simulink model "SmartAgroSense"  (R2026a)
settings: Solver=FixedStepAuto  StopTime=100  FixedStep=0.1
settings Model: Creator=rasul  LastModifiedBy=rasul

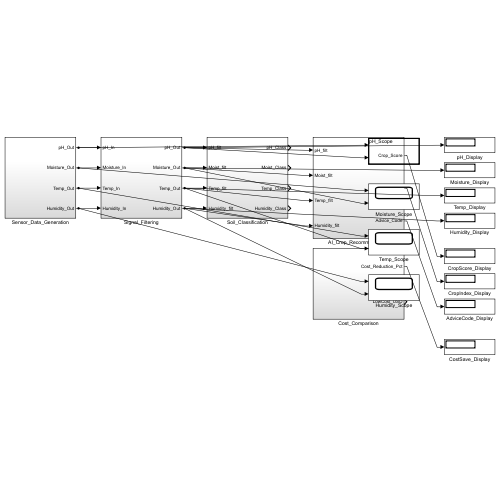
[thumbnail: Simulink's stored preview of the top-level diagram]
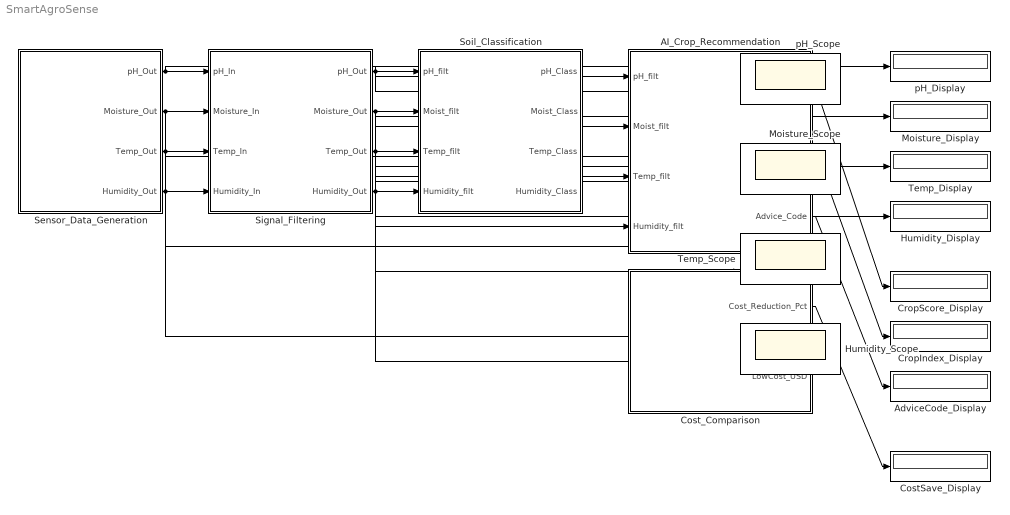
== system SmartAgroSense ==
  AI_Crop_Recommendation : Subsystem
  AdviceCode_Display : Display
  CostSave_Display : Display
  Cost_Comparison : Subsystem
  CropIndex_Display : Display
  CropScore_Display : Display
  Humidity_Display : Display
  Humidity_Scope : Scope  NumInputPorts=2
  Moisture_Display : Display
  Moisture_Scope : Scope  NumInputPorts=2
  Sensor_Data_Generation : Subsystem
  Signal_Filtering : Subsystem
  Soil_Classification : Subsystem
  Temp_Display : Display
  Temp_Scope : Scope  NumInputPorts=2
  pH_Display : Display
  pH_Scope : Scope  NumInputPorts=2
  wires:
  Sensor_Data_Generation/1(pH_Out) -> Signal_Filtering/1(pH_In), pH_Scope/1
  Sensor_Data_Generation/2(Moisture_Out) -> Signal_Filtering/2(Moisture_In), Moisture_Scope/1
  Sensor_Data_Generation/3(Temp_Out) -> Signal_Filtering/3(Temp_In), Temp_Scope/1
  Sensor_Data_Generation/4(Humidity_Out) -> Signal_Filtering/4(Humidity_In), Humidity_Scope/1
  Signal_Filtering/1(pH_Out) -> Soil_Classification/1(pH_filt), AI_Crop_Recommendation/1(pH_filt), pH_Display/1, pH_Scope/2
  Signal_Filtering/2(Moisture_Out) -> Soil_Classification/2(Moist_filt), AI_Crop_Recommendation/2(Moist_filt), Moisture_Display/1, Moisture_Scope/2
  Signal_Filtering/3(Temp_Out) -> Soil_Classification/3(Temp_filt), AI_Crop_Recommendation/3(Temp_filt), Temp_Display/1, Temp_Scope/2
  Signal_Filtering/4(Humidity_Out) -> Soil_Classification/4(Humidity_filt), AI_Crop_Recommendation/4(Humidity_filt), Humidity_Display/1, Humidity_Scope/2
  AI_Crop_Recommendation/1(Crop_Score) -> CropScore_Display/1
  AI_Crop_Recommendation/2(Crop_Index) -> CropIndex_Display/1
  AI_Crop_Recommendation/3(Advice_Code) -> AdviceCode_Display/1
  Cost_Comparison/1(Cost_Reduction_Pct) -> CostSave_Display/1

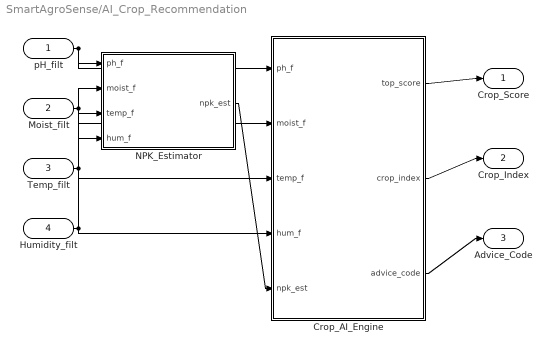
== system SmartAgroSense/AI_Crop_Recommendation ==
  pH_filt : Inport
  Moist_filt : Inport  Port=2
  Temp_filt : Inport  Port=3
  Humidity_filt : Inport  Port=4
  Crop_AI_Engine : MATLAB Function  TreatAsAtomicUnit=on
  NPK_Estimator : MATLAB Function  TreatAsAtomicUnit=on
  Crop_Score : Outport
  Crop_Index : Outport  Port=2
  Advice_Code : Outport  Port=3
  wires:
  pH_filt/1 -> Crop_AI_Engine/1(ph_f), NPK_Estimator/1(ph_f)
  Moist_filt/1 -> Crop_AI_Engine/2(moist_f), NPK_Estimator/2(moist_f)
  Temp_filt/1 -> Crop_AI_Engine/3(temp_f), NPK_Estimator/3(temp_f)
  Humidity_filt/1 -> Crop_AI_Engine/4(hum_f), NPK_Estimator/4(hum_f)
  NPK_Estimator/1(npk_est) -> Crop_AI_Engine/5(npk_est)
  Crop_AI_Engine/1(top_score) -> Crop_Score/1
  Crop_AI_Engine/2(crop_index) -> Crop_Index/1
  Crop_AI_Engine/3(advice_code) -> Advice_Code/1

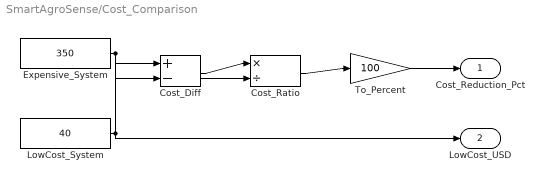
== system SmartAgroSense/Cost_Comparison ==
  Cost_Diff : Sum  Inputs=+-
  Cost_Ratio : Product  Inputs=*/
  Expensive_System : Constant  Value=350
  LowCost_System : Constant  Value=40
  To_Percent : Gain  Gain=100
  Cost_Reduction_Pct : Outport
  LowCost_USD : Outport  Port=2
  wires:
  Expensive_System/1 -> Cost_Diff/1, Cost_Ratio/2
  LowCost_System/1 -> Cost_Diff/2, LowCost_USD/1
  Cost_Diff/1 -> Cost_Ratio/1
  Cost_Ratio/1 -> To_Percent/1
  To_Percent/1 -> Cost_Reduction_Pct/1

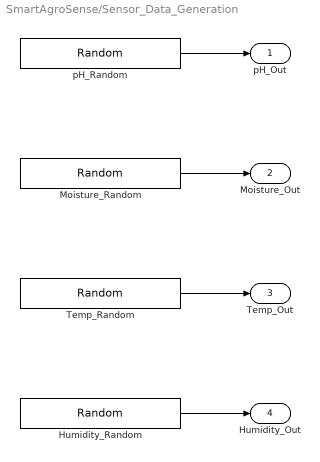
== system SmartAgroSense/Sensor_Data_Generation ==
  Humidity_Random : UniformRandomNumber  Minimum=30  Maximum=95  Seed=1088592771  SampleTime=0.1
  Moisture_Random : UniformRandomNumber  Minimum=10  Maximum=90  Seed=846067018  SampleTime=0.1
  Temp_Random : UniformRandomNumber  Minimum=10  Maximum=40  Seed=366663745  SampleTime=0.1
  pH_Random : UniformRandomNumber  Minimum=4.5  Maximum=8.5  Seed=1463581336  SampleTime=0.1
  pH_Out : Outport
  Moisture_Out : Outport  Port=2
  Temp_Out : Outport  Port=3
  Humidity_Out : Outport  Port=4
  wires:
  pH_Random/1 -> pH_Out/1
  Moisture_Random/1 -> Moisture_Out/1
  Temp_Random/1 -> Temp_Out/1
  Humidity_Random/1 -> Humidity_Out/1

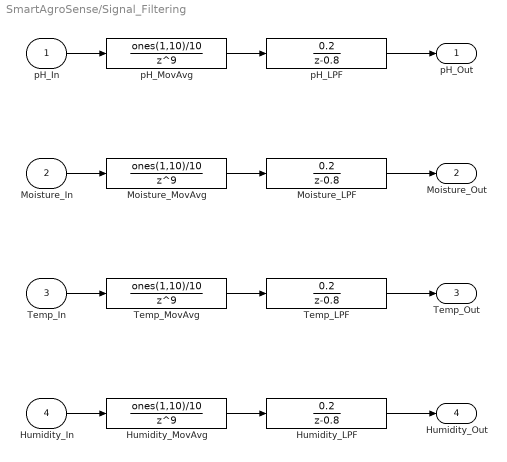
== system SmartAgroSense/Signal_Filtering ==
  pH_In : Inport
  Moisture_In : Inport  Port=2
  Temp_In : Inport  Port=3
  Humidity_In : Inport  Port=4
  Humidity_LPF : DiscreteTransferFcn  Numerator=[0.2]  Denominator=[1, -0.8]  SampleTime=0.1
  Humidity_MovAvg : DiscreteTransferFcn  Numerator=ones(1,10)/10  Denominator=[1 0 0 0 0 0 0 0 0 0]  SampleTime=0.1
  Moisture_LPF : DiscreteTransferFcn  Numerator=[0.2]  Denominator=[1, -0.8]  SampleTime=0.1
  Moisture_MovAvg : DiscreteTransferFcn  Numerator=ones(1,10)/10  Denominator=[1 0 0 0 0 0 0 0 0 0]  SampleTime=0.1
  Temp_LPF : DiscreteTransferFcn  Numerator=[0.2]  Denominator=[1, -0.8]  SampleTime=0.1
  Temp_MovAvg : DiscreteTransferFcn  Numerator=ones(1,10)/10  Denominator=[1 0 0 0 0 0 0 0 0 0]  SampleTime=0.1
  pH_LPF : DiscreteTransferFcn  Numerator=[0.2]  Denominator=[1, -0.8]  SampleTime=0.1
  pH_MovAvg : DiscreteTransferFcn  Numerator=ones(1,10)/10  Denominator=[1 0 0 0 0 0 0 0 0 0]  SampleTime=0.1
  pH_Out : Outport
  Moisture_Out : Outport  Port=2
  Temp_Out : Outport  Port=3
  Humidity_Out : Outport  Port=4
  wires:
  pH_In/1 -> pH_MovAvg/1
  pH_MovAvg/1 -> pH_LPF/1
  pH_LPF/1 -> pH_Out/1
  Moisture_In/1 -> Moisture_MovAvg/1
  Moisture_MovAvg/1 -> Moisture_LPF/1
  Moisture_LPF/1 -> Moisture_Out/1
  Temp_In/1 -> Temp_MovAvg/1
  Temp_MovAvg/1 -> Temp_LPF/1
  Temp_LPF/1 -> Temp_Out/1
  Humidity_In/1 -> Humidity_MovAvg/1
  Humidity_MovAvg/1 -> Humidity_LPF/1
  Humidity_LPF/1 -> Humidity_Out/1

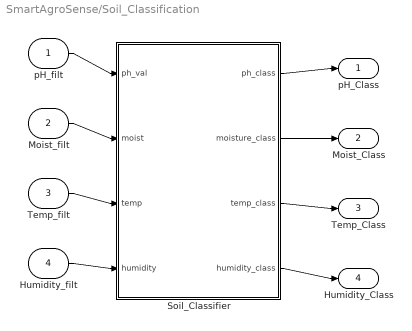
== system SmartAgroSense/Soil_Classification ==
  pH_filt : Inport
  Moist_filt : Inport  Port=2
  Temp_filt : Inport  Port=3
  Humidity_filt : Inport  Port=4
  Soil_Classifier : MATLAB Function  TreatAsAtomicUnit=on
  pH_Class : Outport
  Moist_Class : Outport  Port=2
  Temp_Class : Outport  Port=3
  Humidity_Class : Outport  Port=4
  wires:
  pH_filt/1 -> Soil_Classifier/1(ph_val)
  Moist_filt/1 -> Soil_Classifier/2(moist)
  Temp_filt/1 -> Soil_Classifier/3(temp)
  Humidity_filt/1 -> Soil_Classifier/4(humidity)
  Soil_Classifier/1(ph_class) -> pH_Class/1
  Soil_Classifier/2(moisture_class) -> Moist_Class/1
  Soil_Classifier/3(temp_class) -> Temp_Class/1
  Soil_Classifier/4(humidity_class) -> Humidity_Class/1

== matlab function SmartAgroSense/AI_Crop_Recommendation/NPK_Estimator ==
  data: ph_f input; npk_est output; moist_f input; temp_f input; hum_f input
%% =========================================================================
%  MATLAB Function Block: NPK_Estimator
%  File: npk_estimator_fcn.m
%
%  PURPOSE:
%    Estimate composite NPK availability score (0-100) from filtered
%    pH, moisture, temperature, and humidity readings.
%
%  INPUTS:
%    ph_f    - Filtered pH (4.5 to 8.5)
%    moist_f - Filtered soil moisture % (10 to 90)
%    temp_f  - Filtered temperature C (10 to 40)
%    hum_f   - Filtered humidity % (30 to 95)
%
%  OUTPUT:
%    npk_est - Composite NPK estimate (0 to 100)
%
%  PASTE THIS CODE INTO THE MATLAB FUNCTION BLOCK EDITOR IN SIMULINK
% =========================================================================

function npk_est = npk_estimator(ph_f, moist_f, temp_f, hum_f)
%#codegen

% NPK estimation heuristic:
% - pH near 6.5 generally improves nutrient availability
% - moderate moisture supports uptake
% - temperature/humidity adjust estimated N/P/K availability
ph_penalty = max(0, 1 - abs(ph_f - 6.5) / 2.0);           % 0-1
moist_factor = min(1, max(0, (moist_f - 20) / 50));       % 0-1
temp_factor = max(0, 1 - abs(temp_f - 24) / 16);          % 0-1
hum_factor = min(1, max(0, (hum_f - 35) / 45));           % 0-1

npk_base = 100 * (0.6 * ph_penalty + 0.4 * moist_factor);

n_est = npk_base * (0.85 + 0.25 * moist_factor - 0.10 * (1 - hum_factor));
p_est = npk_base * (0.85 + 0.30 * ph_penalty  - 0.15 * (1 - temp_factor));
k_est = npk_base * (0.90 + 0.20 * ph_penalty  + 0.05 * hum_factor);

n_est = min(100, max(0, n_est));
p_est = min(100, max(0, p_est));
k_est = min(100, max(0, k_est));

npk_est = (n_est + p_est + k_est) / 3;
npk_est = min(100, max(0, npk_est));

end

== matlab function SmartAgroSense/Soil_Classification/Soil_Classifier ==
  data: ph_val input; ph_class output; moist input; temp input; humidity input; moisture_class output; temp_class output; humidity_class output
%% =========================================================================
%  MATLAB Function Block: Soil_Classifier
%  File: soil_classifier_fcn.m
%
%  PURPOSE:
%    Classifies filtered sensor readings into human-readable soil condition
%    categories encoded as integers for display/processing.
%
%  INPUTS:
%    ph_val   - Filtered soil pH (4.5 to 8.5)
%    moist    - Filtered soil moisture % (10 to 90)
%    temp     - Filtered temperature °C (10 to 40)
%    humidity - Filtered air humidity % (30 to 95)
%
%  OUTPUTS:
%    ph_class       - 1=Acidic, 2=Slightly Acidic, 3=Neutral, 4=Alkaline
%    moisture_class - 1=Dry, 2=Moderate, 3=Wet
%    temp_class     - 1=Low, 2=Suitable, 3=High
%    humidity_class - 1=Low, 2=Moderate, 3=High
%
%  PASTE THIS CODE INTO THE MATLAB FUNCTION BLOCK EDITOR IN SIMULINK
% =========================================================================

function [ph_class, moisture_class, temp_class, humidity_class] = ...
    soil_classifier(ph_val, moist, temp, humidity)

%% pH Classification
% Nepal soils range from strongly acidic hill soils to alkaline terai soils
if ph_val < 5.5
    ph_class = 1;     % Strongly Acidic - needs lime
elseif ph_val < 6.5
    ph_class = 2;     % Slightly Acidic - suits most crops
elseif ph_val <= 7.5
    ph_class = 3;     % Neutral - ideal for most Nepal crops
else
    ph_class = 4;     % Alkaline - needs acidifying agents
end

%% Moisture Classification
% Based on volumetric water content equivalents
if moist < 25
    moisture_class = 1;   % Dry - irrigation needed
elseif moist <= 60
    moisture_class = 2;   % Moderate - good for most crops
else
    moisture_class = 3;   % Wet - drainage may be needed
end

%% Temperature Classification
% Based on Nepal's major crop growing seasons
if temp < 15
    temp_class = 1;   % Too Low - only cold-tolerant crops (wheat, barley)
elseif temp <= 32
    temp_class = 2;   % Suitable - rice, maize, vegetables grow well
else
    temp_class = 3;   % Too High - heat stress risk, shade crops
end

%% Humidity Classification
if humidity < 45
    humidity_class = 1;   % Low - drought risk, moisture conservation needed
elseif humidity <= 70
    humidity_class = 2;   % Moderate - balanced for most crops
else
    humidity_class = 3;   % High - disease risk (fungal), good for rice
end

end

== matlab function SmartAgroSense/AI_Crop_Recommendation/Crop_AI_Engine ==
  data: ph_f input; top_score output; moist_f input; temp_f input; hum_f input; npk_est input; crop_index output; advice_code output
%% =========================================================================
%  MATLAB Function Block: Crop_AI_Engine
%  File: crop_ai_engine_fcn.m
%
%  PURPOSE:
%    Rule-based AI engine that calculates suitability scores for 8 Nepal
%    crops based on filtered soil and environment sensor readings.
%    Selects the top crop and provides a soil improvement advice code.
%
%  CROPS SUPPORTED (index mapping):
%    1 = Rice      | 2 = Maize    | 3 = Wheat
%    4 = Mustard   | 5 = Potato   | 6 = Tomato
%    7 = Lentil    | 8 = Millet
%
%  INPUTS:
%    ph_f    - Filtered pH (4.5 - 8.5)
%    moist_f - Filtered moisture % (10 - 90)
%    temp_f  - Filtered temperature °C (10 - 40)
%    hum_f   - Filtered humidity % (30 - 95)
%    npk_est - Estimated NPK composite score (0-100)
%
%  OUTPUTS:
%    top_score   - Suitability score of best crop (0-100)
%    crop_index  - Index of best crop (1-8, see above)
%    advice_code - Soil improvement advice code (1-6, see legend below)
%
%  ADVICE CODE LEGEND:
%    1 = Add lime to raise pH
%    2 = Add sulfur/organic matter to lower pH
%    3 = Irrigate - soil too dry
%    4 = Improve drainage - soil too wet
%    5 = Add NPK fertilizer - low fertility
%    6 = Soil conditions are good - maintain practices
%
%  PASTE THIS CODE INTO THE MATLAB FUNCTION BLOCK EDITOR IN SIMULINK
% =========================================================================

function [top_score, crop_index, advice_code] = ...
    crop_ai_engine(ph_f, moist_f, temp_f, hum_f, npk_est)

%% -----------------------------------------------------------------------
%  CROP REQUIREMENT TABLE
%  Each row: [pH_min, pH_opt_lo, pH_opt_hi, pH_max,
%             moist_min, moist_opt_lo, moist_opt_hi, moist_max,
%             temp_min, temp_opt_lo, temp_opt_hi, temp_max,
%             hum_min, hum_opt_lo, hum_opt_hi, hum_max,
%             npk_min]
% -----------------------------------------------------------------------

% Crop: Rice
rice     = [5.0, 6.0, 7.0, 8.0,  50, 65, 80, 90,  20, 25, 35, 40,  60, 70, 90, 95,  60];
% Crop: Maize
maize    = [5.5, 6.0, 7.0, 8.0,  30, 45, 65, 80,  18, 22, 32, 38,  40, 55, 80, 90,  55];
% Crop: Wheat
wheat    = [5.5, 6.0, 7.0, 8.0,  25, 40, 60, 70,  10, 15, 22, 28,  35, 50, 70, 85,  50];
% Crop: Mustard
mustard  = [5.5, 6.0, 7.0, 7.5,  20, 35, 55, 70,  10, 15, 25, 30,  30, 45, 65, 80,  40];
% Crop: Potato
potato   = [4.8, 5.5, 6.5, 7.0,  40, 55, 70, 80,  14, 18, 24, 28,  45, 60, 80, 90,  65];
% Crop: Tomato
tomato   = [5.5, 6.0, 6.8, 7.5,  35, 50, 65, 75,  18, 22, 28, 35,  40, 55, 75, 85,  60];
% Crop: Lentil
lentil   = [5.8, 6.5, 7.5, 8.0,  20, 35, 50, 65,  12, 18, 25, 30,  30, 45, 65, 75,  35];
% Crop: Millet
millet   = [5.0, 5.5, 6.5, 7.5,  20, 35, 55, 70,  20, 25, 35, 40,  30, 45, 70, 85,  30];

% Stack into matrix [8 x 17]
cropTable = [rice; maize; wheat; mustard; potato; tomato; lentil; millet];
nCrops = 8;

%% -----------------------------------------------------------------------
%  SUITABILITY SCORE CALCULATION
%  For each parameter, score = 0-100 based on trapezoidal membership:
%    Score = 100 if value in [opt_lo, opt_hi]
%    Score = 0   if value < min or value > max
%    Linearly interpolated in between
% -----------------------------------------------------------------------

scores = zeros(1, nCrops);

for c = 1:nCrops
    req = cropTable(c, :);
    
    % pH score
    ph_score = trapezoid_score(ph_f, req(1), req(2), req(3), req(4));
    
    % Moisture score
    m_score = trapezoid_score(moist_f, req(5), req(6), req(7), req(8));
    
    % Temperature score
    t_score = trapezoid_score(temp_f, req(9), req(10), req(11), req(12));
    
    % Humidity score
    h_score = trapezoid_score(hum_f, req(13), req(14), req(15), req(16));
    
    % NPK score (simple threshold)
    if npk_est >= req(17)
        npk_score = 100;
    elseif npk_est >= req(17) * 0.5
        npk_score = 100 * (npk_est - req(17)*0.5) / (req(17)*0.5);
    else
        npk_score = 0;
    end
    
    % Weighted composite score
    % pH and temperature are critical -> higher weight
    scores(c) = 0.30 * ph_score + ...
                0.25 * m_score  + ...
                0.25 * t_score  + ...
                0.10 * h_score  + ...
                0.10 * npk_score;
end

%% -----------------------------------------------------------------------
%  SELECT BEST CROP
% -----------------------------------------------------------------------
[top_score, crop_index] = max(scores);
top_score = round(top_score);   % Round to integer for display

%% -----------------------------------------------------------------------
%  GENERATE ADVICE CODE
% -----------------------------------------------------------------------
if ph_f < 5.5
    advice_code = 1;    % Add lime to raise pH
elseif ph_f > 7.8
    advice_code = 2;    % Add sulfur/organic matter to lower pH
elseif moist_f < 25
    advice_code = 3;    % Irrigate
elseif moist_f > 75
    advice_code = 4;    % Improve drainage
elseif npk_est < 35
    advice_code = 5;    % Add NPK fertilizer
else
    advice_code = 6;    % Soil conditions are good
end

end

%% -----------------------------------------------------------------------
%  HELPER: Trapezoidal Membership Function
%  Returns score 0-100
%    0   if x < a (below minimum)
%    0-100 ramping up from a to b
%    100  if b <= x <= c (optimal range)
%    100-0 ramping down from c to d
%    0   if x > d (above maximum)
% -----------------------------------------------------------------------
function score = trapezoid_score(x, a, b, c, d)
    if x <= a || x >= d
        score = 0;
    elseif x >= b && x <= c
        score = 100;
    elseif x > a && x < b
        score = 100 * (x - a) / (b - a);
    else  % x > c && x < d
        score = 100 * (d - x) / (d - c);
    end
end
